simulink model "marine_otter_velocity"  (R2024a)
settings: Solver=FixedStepAuto  StartTime=0.0  StopTime=10.0  FixedStep=0.05  RelTol=1e-3
PostLoadFcn:
  | on_model_load
InitFcn:
  | on_model_start
StopFcn:
  | on_simulation_done
undefined symbols (not defined in the file or in its folder): ActiveScenario
libraries: data_driven_lib_ctl x2, marine_lib_sys x2
PostSaveFcn:
  | on_model_save
settings Model: Creator=luka  LastModifiedBy=luka

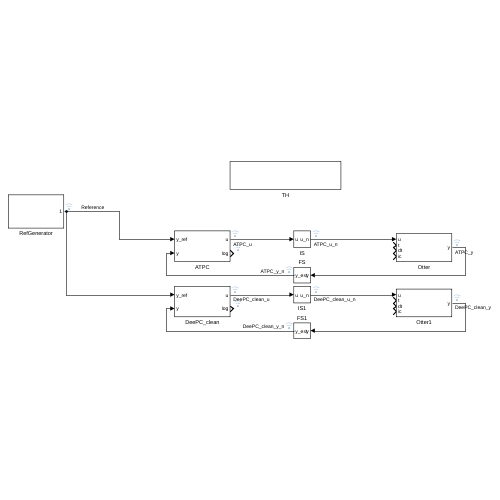
[thumbnail: Simulink's stored preview of the top-level diagram]
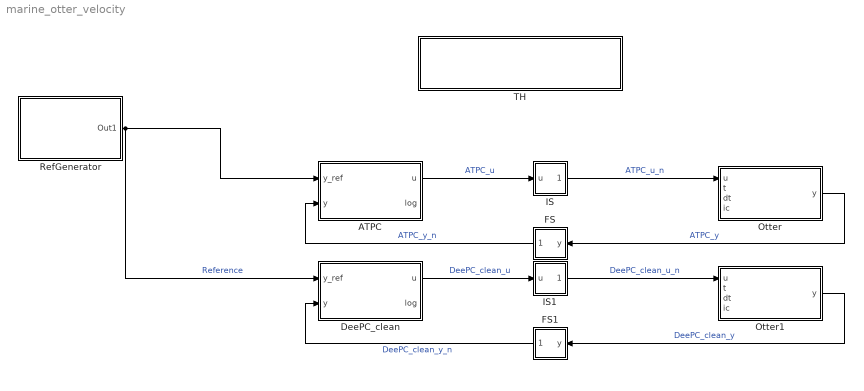
== system marine_otter_velocity ==
  ATPC : Subsystem  Tag=__cs_template;__cs_comptype:ctl
      mask DialogControl ParameterGroupVar Prompt: Params
  DeePC_clean : Subsystem  Tag=__cs_template;__cs_comptype:ctl
      mask DialogControl ParameterGroupVar Prompt: Params
  FS : Subsystem
  FS1 : Subsystem
  IS : Subsystem
  IS1 : Subsystem
  Otter : Subsystem  Tag=__cs_template;__cs_comptype:sys
      mask DialogControl ParameterGroupVar Prompt: Params
  Otter1 : Subsystem  Tag=__cs_template;__cs_comptype:sys
      mask DialogControl ParameterGroupVar Prompt: Params
  RefGenerator : Subsystem  mask{experiment=P1}
      settings: OpenFcn=on_reference_generator_open();
      mask TypeOptions experiment: P1
      mask Callback experiment: on_experiment_select;
      mask DialogControl DescGroupVar Prompt: Select experiment
  TH : Subsystem
      mask DialogControl ParameterGroupVar Prompt: Params
  wires:
  ATPC/1(u) -> IS/1(u)  "ATPC_u"
  IS/1(u_n) -> Otter/1(u)  "ATPC_u_n"
  Otter/1(y) -> FS/1(y)  "ATPC_y"
  FS/1(y_est) -> ATPC/2(y)  "ATPC_y_n"
  RefGenerator/1(Out1) -> ATPC/1(y_ref), DeePC_clean/1(y_ref)  "Reference"
  DeePC_clean/1(u) -> IS1/1(u)  "DeePC_clean_u"
  IS1/1(u_n) -> Otter1/1(u)  "DeePC_clean_u_n"
  Otter1/1(y) -> FS1/1(y)  "DeePC_clean_y"
  FS1/1(y_est) -> DeePC_clean/2(y)  "DeePC_clean_y_n"

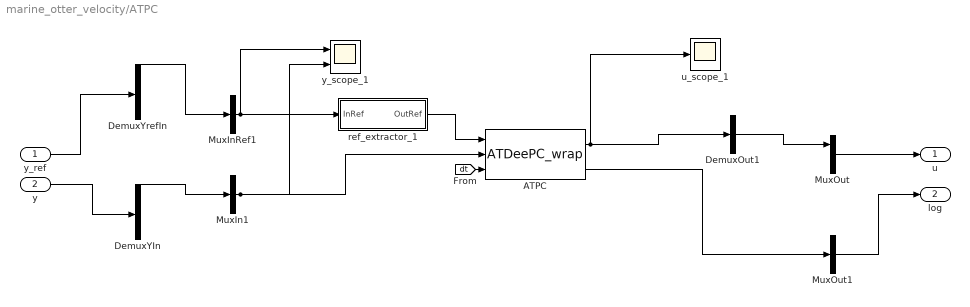
== system marine_otter_velocity/ATPC ==
  y_ref : Inport  PortDimensions=12
  y : Inport  Port=2  PortDimensions=12
  ATPC : data_driven_lib_ctl/ATDeePC_wrap  Tag=controller;__cs_comptype:ctl;__cs_compimpl:slx;  trajectory_T=0  data=0  db_params=0  deepc_params=0  iid__=[54 100 98 51 99 102 48 101 45 52 54 50 100 45 52 99 51 53 45 97 100 52 51 45 56 49 99 101 49 102 55 97 102 48 52 55]  pid__=[65 84 68 101 101 80 67 95 119 114 97 112 58 100 97 116 97 95 100 114 105 118 101 110 95 108 105 98]  params=marine_otter_velocity_params.ctl.ATPC  params_struct_name=marine_otter_velocity_params.ctl.ATPC
  DemuxOut1 : Demux  Outputs=1
  DemuxYIn : Demux  Outputs=12
  DemuxYrefIn : Demux  Outputs=12
  MuxIn1 : Mux  Inputs=1
  MuxInRef1 : Mux  Inputs=1
  MuxOut : Mux  Inputs=2
  MuxOut1 : BusCreator  Inputs=1
  ref_extractor_1 : Subsystem
  u_scope_1 : Scope
  y_scope_1 : Scope  NumInputPorts=2
  u : Outport  PortDimensions=2
  log : Outport  Port=2
  wires:
  [dt] -> ATPC/3
  y/1 -> DemuxYIn/1
  y_ref/1 -> DemuxYrefIn/1
  MuxOut/1 -> u/1
  MuxOut1/1 -> log/1
  MuxInRef1/1 -> ref_extractor_1/1(InRef), y_scope_1/1
  ref_extractor_1/1(OutRef) -> ATPC/1
  MuxIn1/1 -> ATPC/2, y_scope_1/2
  ATPC/1 -> DemuxOut1/1, u_scope_1/1
  ATPC/2 -> MuxOut1/1
  DemuxYIn/1 -> MuxIn1/1
  DemuxYrefIn/1 -> MuxInRef1/1
  DemuxOut1/1 -> MuxOut/1

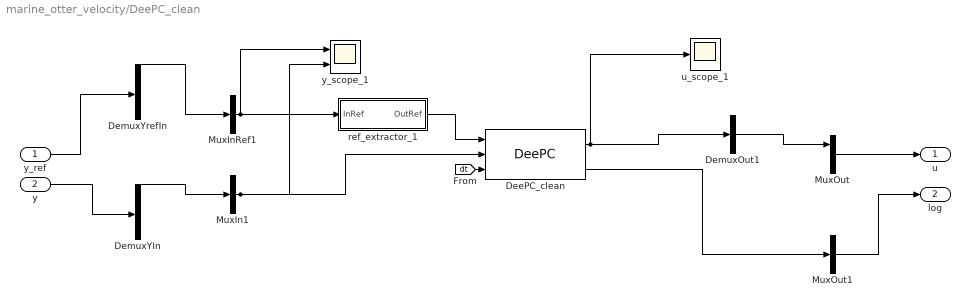
== system marine_otter_velocity/DeePC_clean ==
  y_ref : Inport  PortDimensions=12
  y : Inport  Port=2  PortDimensions=12
  DeePC_clean : data_driven_lib_ctl/DeePC  Tag=__cs_comptype:ctl;__cs_compimpl:mat;  iid__=[102 52 49 101 102 57 101 52 45 98 97 51 52 45 52 49 54 99 45 56 52 98 54 45 55 55 57 52 57 53 54 97 51 99 48 52]  pid__=[68 101 101 80 67 58 100 97 116 97 95 100 114 105 118 101 110 95 108 105 98]  params=marine_otter_velocity_params.ctl.DeePC_clean  LogEntryType=DeePC_LT  data=DeePC_data  ParamsType=DeePC_PT  DataType=DeePC_DT  u_ic=0
  DemuxOut1 : Demux  Outputs=1
  DemuxYIn : Demux  Outputs=12
  DemuxYrefIn : Demux  Outputs=12
  MuxIn1 : Mux  Inputs=1
  MuxInRef1 : Mux  Inputs=1
  MuxOut : Mux  Inputs=2
  MuxOut1 : BusCreator  Inputs=1
  ref_extractor_1 : Subsystem
  u_scope_1 : Scope
  y_scope_1 : Scope  NumInputPorts=2
  u : Outport  PortDimensions=2
  log : Outport  Port=2
  wires:
  [dt] -> DeePC_clean/3
  y/1 -> DemuxYIn/1
  y_ref/1 -> DemuxYrefIn/1
  MuxOut/1 -> u/1
  MuxOut1/1 -> log/1
  MuxInRef1/1 -> ref_extractor_1/1(InRef), y_scope_1/1
  ref_extractor_1/1(OutRef) -> DeePC_clean/1
  MuxIn1/1 -> DeePC_clean/2, y_scope_1/2
  DeePC_clean/1 -> DemuxOut1/1, u_scope_1/1
  DeePC_clean/2 -> MuxOut1/1
  DemuxYIn/1 -> MuxIn1/1
  DemuxYrefIn/1 -> MuxInRef1/1
  DemuxOut1/1 -> MuxOut/1

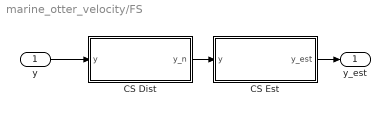
== system marine_otter_velocity/FS ==
  y : Inport
  CS Dist : Subsystem
      mask DialogControl ParameterGroupVar Prompt: Params
  CS Est : Subsystem
      mask DialogControl ParameterGroupVar Prompt: Params
  y_est : Outport
  wires:
  CS Est/1(y_est) -> y_est/1
  CS Dist/1(y_n) -> CS Est/1(y)
  y/1 -> CS Dist/1(y)

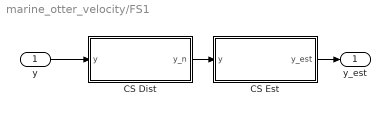
== system marine_otter_velocity/FS1 ==
  y : Inport
  CS Dist : Subsystem
      mask DialogControl ParameterGroupVar Prompt: Params
  CS Est : Subsystem
      mask DialogControl ParameterGroupVar Prompt: Params
  y_est : Outport
  wires:
  CS Est/1(y_est) -> y_est/1
  CS Dist/1(y_n) -> CS Est/1(y)
  y/1 -> CS Dist/1(y)

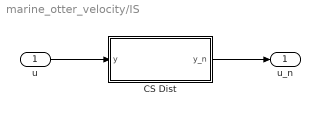
== system marine_otter_velocity/IS ==
  u : Inport
  CS Dist : Subsystem
      mask DialogControl ParameterGroupVar Prompt: Params
  u_n : Outport
  wires:
  CS Dist/1(y_n) -> u_n/1
  u/1 -> CS Dist/1(y)

== system marine_otter_velocity/IS1 ==
  u : Inport
  CS Dist : Subsystem
      mask DialogControl ParameterGroupVar Prompt: Params
  u_n : Outport
  wires:
  CS Dist/1(y_n) -> u_n/1
  u/1 -> CS Dist/1(y)

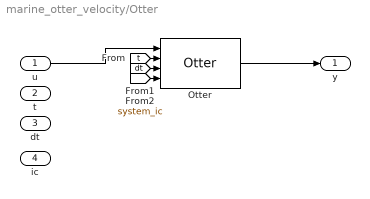
== system marine_otter_velocity/Otter ==
  u : Inport
  t : Inport  Port=2
  dt : Inport  Port=3
  ic : Inport  Port=4
  Otter : marine_lib_sys/Otter  Tag=system;__cs_slx_sys;__cs_comptype:sys;__cs_compimpl:slx;  payload_mass=0  payload_location=[0,0, 0]  current_speed=0  current_direction=0  out_gain=1  iid__=[52 97 48 100 49 48 49 48 45 52 53 52 57 45 52 100 53 49 45 98 51 97 53 45 54 48 50 101 55 99 57 51 50 98 52 53]  pid__=[79 116 116 101 114 58 109 97 114 105 110 101 95 108 105 98]  params=ActiveScenario.SystemParams  params_struct_name=marine_otter_velocity_params.sys.Otter
  y : Outport
  wires:
  u/1 -> Otter/1
  Otter/1 -> y/1
  [t] -> Otter/2
  [dt] -> Otter/3
  [system_ic] -> Otter/4

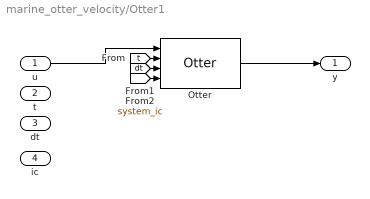
== system marine_otter_velocity/Otter1 ==
  u : Inport
  t : Inport  Port=2
  dt : Inport  Port=3
  ic : Inport  Port=4
  Otter : marine_lib_sys/Otter  Tag=system;__cs_slx_sys;__cs_comptype:sys;__cs_compimpl:slx;  payload_mass=0  payload_location=[0,0, 0]  current_speed=0  current_direction=0  out_gain=1  iid__=[52 97 48 100 49 48 49 48 45 52 53 52 57 45 52 100 53 49 45 98 51 97 53 45 54 48 50 101 55 99 57 51 50 98 52 53]  pid__=[79 116 116 101 114 58 109 97 114 105 110 101 95 108 105 98]  params=ActiveScenario.SystemParams  params_struct_name=marine_otter_velocity_params.sys.Otter
  y : Outport
  wires:
  u/1 -> Otter/1
  Otter/1 -> y/1
  [t] -> Otter/2
  [dt] -> Otter/3
  [system_ic] -> Otter/4

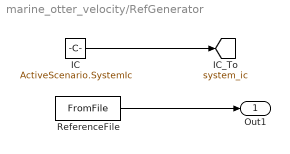
== system marine_otter_velocity/RefGenerator ==
  IC : Constant  Value=ActiveScenario.SystemIc
  ReferenceFile : FromFile  SampleTime=0
  Out1 : Outport
  tag scope: system_ic=global
  wires:
  IC/1 -> [system_ic]
  ReferenceFile/1 -> Out1/1

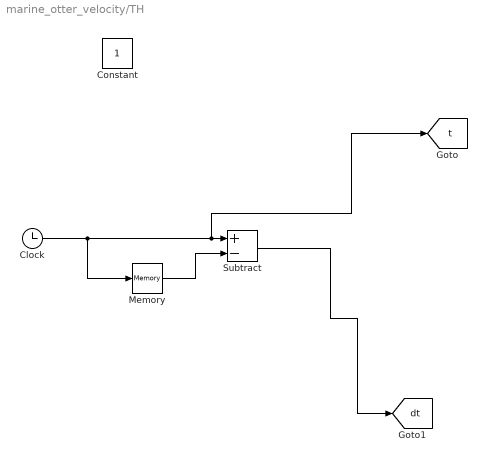
== system marine_otter_velocity/TH ==
  Clock : Clock
  Constant : Constant
  Memory : Memory
  Subtract : Sum  Inputs=+-
  tag scope: dt=global, t=global
  wires:
  Subtract/1 -> [dt]
  Memory/1 -> Subtract/2
  Clock/1 -> Memory/1, Subtract/1, [t]

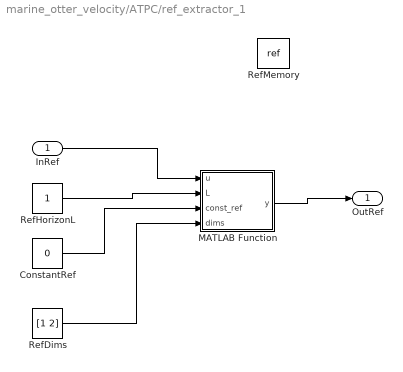
== system marine_otter_velocity/ATPC/ref_extractor_1 ==
  InRef : Inport
  ConstantRef : Constant  Value=0
  MATLAB Function : MATLAB Function  TreatAsAtomicUnit=on
  RefDims : Constant  Value=[1 2]
  RefHorizonL : Constant
  RefMemory : DataStoreMemory  DataStoreName=ref  WriteAfterWriteMsg=warning  ShowAdditionalParam=off  OutDataTypeStr=double
  OutRef : Outport
  wires:
  ConstantRef/1 -> MATLAB Function/3(const_ref)
  RefDims/1 -> MATLAB Function/4(dims)
  RefHorizonL/1 -> MATLAB Function/2(L)
  InRef/1 -> MATLAB Function/1(u)
  MATLAB Function/1(y) -> OutRef/1

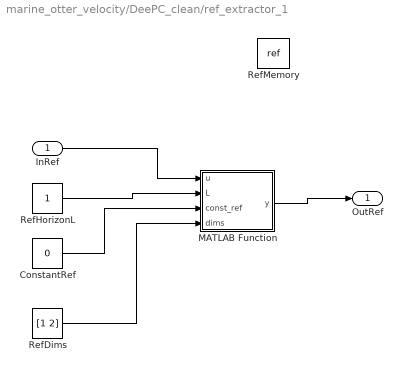
== system marine_otter_velocity/DeePC_clean/ref_extractor_1 ==
  InRef : Inport
  ConstantRef : Constant  Value=0
  MATLAB Function : MATLAB Function  TreatAsAtomicUnit=on
  RefDims : Constant  Value=[1 2]
  RefHorizonL : Constant
  RefMemory : DataStoreMemory  DataStoreName=ref  WriteAfterWriteMsg=warning  ShowAdditionalParam=off  OutDataTypeStr=double
  OutRef : Outport
  wires:
  ConstantRef/1 -> MATLAB Function/3(const_ref)
  RefDims/1 -> MATLAB Function/4(dims)
  RefHorizonL/1 -> MATLAB Function/2(L)
  InRef/1 -> MATLAB Function/1(u)
  MATLAB Function/1(y) -> OutRef/1

== system marine_otter_velocity/FS/CS Dist ==
  y : Inport
  Gain : Gain
  y_n : Outport
  wires:
  Gain/1 -> y_n/1
  y/1 -> Gain/1

== system marine_otter_velocity/FS/CS Est ==
  y : Inport
  Gain : Gain
  y_est : Outport
  wires:
  y/1 -> Gain/1
  Gain/1 -> y_est/1

== system marine_otter_velocity/FS1/CS Dist ==
  y : Inport
  Gain : Gain
  y_n : Outport
  wires:
  Gain/1 -> y_n/1
  y/1 -> Gain/1

== system marine_otter_velocity/FS1/CS Est ==
  y : Inport
  Gain : Gain
  y_est : Outport
  wires:
  y/1 -> Gain/1
  Gain/1 -> y_est/1

== system marine_otter_velocity/IS/CS Dist ==
  y : Inport
  Gain : Gain
  y_n : Outport
  wires:
  y/1 -> Gain/1
  Gain/1 -> y_n/1

== system marine_otter_velocity/IS1/CS Dist ==
  y : Inport
  Gain : Gain
  y_n : Outport
  wires:
  y/1 -> Gain/1
  Gain/1 -> y_n/1

== matlab function marine_otter_velocity/DeePC_clean/ref_extractor_1/MATLAB Function ==
  settings: updateMethod=DISCRETE
  data: u input; L input; const_ref input; dims input; y output; ref data_store_memory; GlobalReference parameter
function y = fcn(u, L, const_ref, dims, GlobalReference)

persistent cnt
global ref

if isempty(cnt)
    cnt = 0;
end

if GlobalReference == 0
    y = repmat(u', 1);
    return;
end


cnt = cnt+1;

horizon_end = cnt+L-1;
if L > 1 
   if horizon_end > length(GlobalReference)
        if size(ref, 1) == size(u, 1)
            y = permute(ref, [2, 1]);
        else
            y = ref;
        end       
        return
   end

   if size(ref, 1) == size(u, 1)
      
      if const_ref == 0
        ref(:, :) = GlobalReference(cnt:horizon_end, dims)';
      else
        ref(:, :) = repmat(GlobalReference(cnt, dims)', 1, L);
      end
      y = permute(ref, [2, 1]);
   else
      if const_ref == 0
        ref(1:L, :) = GlobalReference(cnt:horizon_end, dims);
      else
        ref(1:L, :) = repmat(GlobalReference(cnt, dims), L, 1);
      end
      y = ref;
   end
else
   if size(ref, 1) == size(u, 1)
       ref = u;
       y = permute(ref, [2, 1]);
   else
      ref(1, :) = u';
      y = ref;
   end
end

== matlab function marine_otter_velocity/ATPC/ref_extractor_1/MATLAB Function ==
  settings: updateMethod=DISCRETE
  data: u input; L input; const_ref input; dims input; y output; ref data_store_memory; GlobalReference parameter
function y = fcn(u, L, const_ref, dims, GlobalReference)

persistent cnt
global ref

if isempty(cnt)
    cnt = 0;
end

if GlobalReference == 0
    y = repmat(u', 1);
    return;
end


cnt = cnt+1;

horizon_end = cnt+L-1;
if L > 1 
   if horizon_end > length(GlobalReference)
        if size(ref, 1) == size(u, 1)
            y = permute(ref, [2, 1]);
        else
            y = ref;
        end       
        return
   end

   if size(ref, 1) == size(u, 1)
      
      if const_ref == 0
        ref(:, :) = GlobalReference(cnt:horizon_end, dims)';
      else
        ref(:, :) = repmat(GlobalReference(cnt, dims)', 1, L);
      end
      y = permute(ref, [2, 1]);
   else
      if const_ref == 0
        ref(1:L, :) = GlobalReference(cnt:horizon_end, dims);
      else
        ref(1:L, :) = repmat(GlobalReference(cnt, dims), L, 1);
      end
      y = ref;
   end
else
   if size(ref, 1) == size(u, 1)
       ref = u;
       y = permute(ref, [2, 1]);
   else
      ref(1, :) = u';
      y = ref;
   end
end
